simulink model "SI_Model_Manual"  (R2017b)
settings: Solver=VariableStepAuto  StartTime=0.0  StopTime=500  RelTol=1e-3
model workspace (MAT data in the model file):
  DOWN_TABLE = [0  5  20  35; 0  5  20  35; 0  5  25  40; 0  5  30  50; 0  30  50  80; 0  30  50  80]
  DOWN_TH_BP = [0; 0.05; 0.4; 0.5; 0.9; 1]
  TWAIT = 2
  UP_TABLE = [10  30  50  1000000; 10  30  50  1000000; 15  30  50  1000000; 23  41  60  1000000; 40  70  100  1000000; 40  70  100  1000000]
  UP_TH_BP = [0; 0.25; 0.35; 0.5; 0.9; 1]
  Var1 = 0
  clutchRise = 0.1
  eff_tor_rad = 0.4
  engagement_area = 0.0025
  fric_coeff = 0.5
  gear1 = 3.07
  gear2 = 1.913
  gear3 = 1.258
  gear4 = 0.943
  gear5 = 0.763
  gearx = 4.529
  num_fric_surf = 6
  p0 = 2000000
  peak_normal = 0.55
  pressThresh = 0.05
  v0 = 0
  velTol = 0.001
values from neighbouring files (symbols this model uses):
  HEV_Param =     [DataWorkSpace.mat]
libraries: sdl_lib x17, nesl_utility x15, fl_lib x13, drivecyclelib x1, simulink x1
settings Model: PauseTimes=60  Creator=Charlie  LastModifiedBy=Charlie
settings SolverCC: ZeroCrossAlgorithm=Adaptive  AlgebraicLoopSolver=LineSearch
settings SimscapeCC: SimscapeLogType=all  SimscapeLogSimulationStatistics=on  SimscapeLogOpenViewer=on

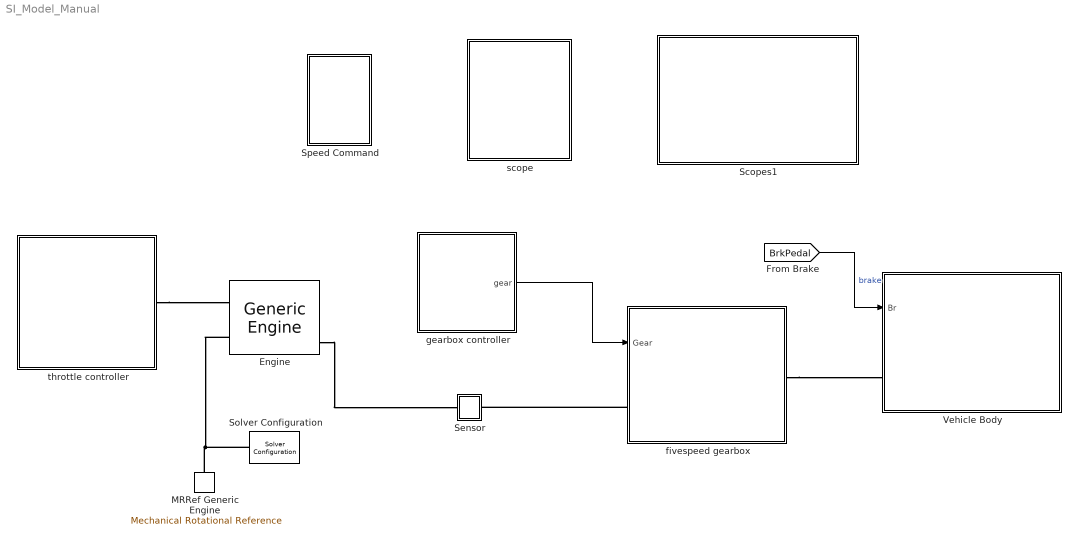
== system SI_Model_Manual ==
  Engine : sdl_lib/Engines/Generic Engine  model_parameterization=1  engine_type=1  P_max=52 kW  w_P_max=6000 rpm  w_max=7000 rpm  w_min=500 rpm  w_tab=[ 500 1000 2e+3 3e+3 4e+3 5e+3 6e+3 7e+3 ] rpm  trq_tab=[ 40 41 42 46 49 42 41 40 ] N*m  pwr_tab=[ 2e+4 4e+4 7.8e+4 1.2e+5 1.45e+5 1.48e+5 1.25e+5 6e+4 ] W  interp_method=1  model_inertia=1  inertia=HEV_Param.ICE.Shaft_Inertia kg*m^2  initial_velocity=800 rpm  model_time_constant=1  time_constant=0.01 s  T0=0  w_thr=100 rpm  idle_speed=1  idle_speed_reference=800 rpm  tau_controller=0.01 s  idle_w_thr=1 rpm  redline=0  redline_speed=7000 rpm  tau_redline=1 s  redline_w_thr=1 rpm  fc_model=1  fc_per_rev=6.2 mg/rev  displaced_volume=400 cm^3  rev_per_cycle=2  fc_w_tab=[ 1000 2e+3 3e+3 4e+3 5e+3 6e+3 ] rpm  fc_trq_tab=[ 0 80 160 200 240 320 360 400 ] N*m  fc_tab=[ 0.5 0.9 1.4 1.6 1.9 2.7 3.4 4.4; 1 1.7 2.7 3.1 3.6 5 6 7.4; 1.4 2.7 4 4.8 5.6 7.5 8.5 10.5; 2 3.6 5.8 6.7 8 10.4 11.7 13.3; 2.5 4.8 7.9 9.4 10.8 14 16.2 18.6; 3.1 6 10.3 11.9 13.8 18.4 22 26.5 ] g/s  bmep_tab=[ 0 250 500 625 750 1000 1.15e+3 1.25e+3 ] kPa  bsfc_tab=[ 410 380 300 280 270 290 320 380; 410 370 290 270 260 270 285 320; 415 380 290 275 265 270 270 300; 420 390 310 290 285 280 280 285; 430 410 340 320 310 300 310 320; 450 430 370 340 330 330 350 380 ] g/hr/kW  fc_interp_method=1
      settings: SourceProductName=Simscape Driveline  SourceProductBaseCode=LD
  MRRef Generic Engine : fl_lib/Mechanical/Rotational Elements/Mechanical Rotational Reference
  Scopes1 : Subsystem  mask(Data Acquisition){}
      mask Display: image('D:\Matlab\Powertrain\Plot\Fuel_Tank.jpg');
  Sensor : Subsystem
      mask Display: disp('S');
  Solver Configuration : nesl_utility/Solver Configuration  PhysicalDomain=network_engine_domain  SubClassName=solver  LeftPortType=input  RightPortType=generic  Accelerate=off  Tones=[]  Harmonics=[]  SimulateNoise=off  Profile=off  UseLocalSampling=off  EnableSwitchedLinearOptims=on  FrequencyDomain=off  UseCCode=off  RelTol=0.001  AbsTol=1e-06  MinStep=1e-09  ToWorkspace=off  RevertToSquareIcSolve=off  NumHomotopyIterations=100  PhasorMode=off  PhasorModeNumHarmonics=1  DoDC=off  ResidualTolerance=1e-9  UseLocalSolver=off  LocalSolverChoice=NE_BACKWARD_EULER_ADVANCER  LocalSolverSampleTime=.01  DoFixedCost=off  MaxNonlinIter=3  MaxModeIter=2  LinearAlgebra=Sparse  DelaysMemoryBudget=1024  AutomaticFiltering=on  FilteringTimeConstant=0.001
  Speed Command : Subsystem
  Vehicle Body : Subsystem  Tag=PublishSubsystem
      mask Display: image('D:\Matlab\Powertrain\Plot\smart_fortw.jpg');
  fivespeed gearbox : Subsystem  Tag=PublishSubsystem
      mask Display: image(imread('sdl_transmission_5spd_schematic.jpg'),'center');
  gearbox controller : Subsystem
  scope : Subsystem
  throttle controller : Subsystem
      mask Display: image('D:\Matlab\Powertrain\Plot\throttle.JPG');
  wires:
  [BrkPedal] -> Vehicle Body/1(Br)  "brake"
  gearbox controller/1(gear) -> fivespeed gearbox/1(Gear)
  connections:
  MRRef Generic Engine/LConn1 -- Engine/LConn2 -- Solver Configuration/RConn1
  fivespeed gearbox/LConn1 -- Sensor/RConn1
  fivespeed gearbox/RConn1 -- Vehicle Body/LConn1
  Engine/RConn3 -- Sensor/LConn1
  throttle controller/RConn1 -- Engine/LConn1

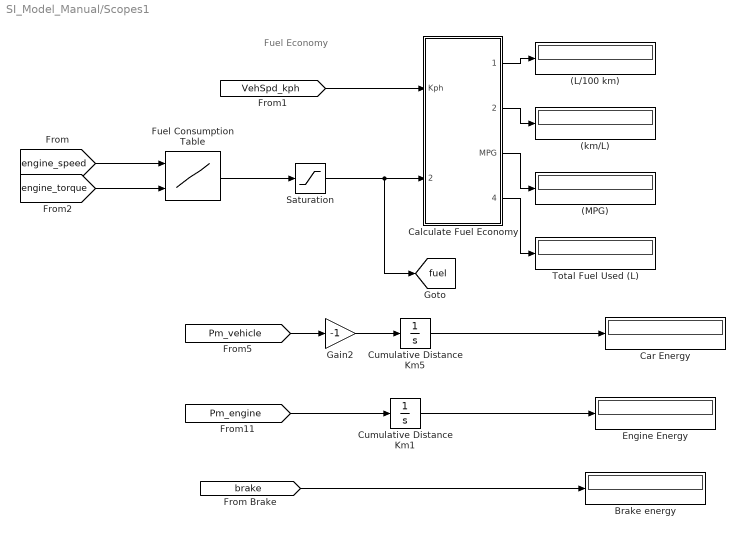
== system SI_Model_Manual/Scopes1 ==
  note: Fuel Economy
  (L/100 km) : Display
      settings: Decimation=decimation
  (MPG) : Display
      settings: Decimation=decimation
  (km/L) : Display
      settings: Decimation=decimation
  Brake energy : Display
      settings: Decimation=decimation
  Calculate Fuel Economy : Subsystem
  Car Energy : Display
      settings: Decimation=decimation
  Cumulative Distance Km1 : Integrator  InitialCondition=eps
  Cumulative Distance Km5 : Integrator  InitialCondition=eps
  Engine Energy : Display
      settings: Decimation=decimation
  Fuel Consumption Table : Lookup2D  RowIndex=HEV_Param.ICE.FC.Speed_Vector  ColumnIndex=HEV_Param.ICE.FC.Torque_Vector  Table=HEV_Param.ICE.FC.Consumption_Table
  Gain2 : Gain  Gain=-1
  Saturation : Saturate  UpperLimit=inf  LowerLimit=0
  Total Fuel Used (L) : Display
      settings: Decimation=decimation
  tag scope: fuel=global
  wires:
  Calculate Fuel Economy/1(Liter/100Km) -> (L/100 km)/1
  Calculate Fuel Economy/3(MPG) -> (MPG)/1
  [VehSpd_kph] -> Calculate Fuel Economy/1(Kph)
  Calculate Fuel Economy/4(Fuel Used (L)) -> Total Fuel Used (L)/1
  Calculate Fuel Economy/2(Km/Liter) -> (km/L)/1
  Fuel Consumption Table/1 -> Saturation/1
  [engine_speed] -> Fuel Consumption Table/1
  [engine_torque] -> Fuel Consumption Table/2
  Gain2/1 -> Cumulative Distance Km5/1
  Cumulative Distance Km5/1 -> Car Energy/1
  [Pm_vehicle] -> Gain2/1
  [Pm_engine] -> Cumulative Distance Km1/1
  Cumulative Distance Km1/1 -> Engine Energy/1
  [brake] -> Brake energy/1
  Saturation/1 -> [fuel], Calculate Fuel Economy/2(Fuel Flow g/s)

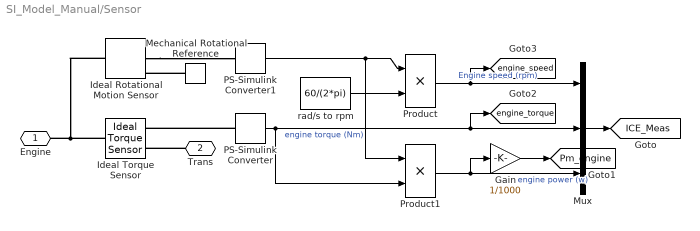
== system SI_Model_Manual/Sensor ==
  Gain : Gain  Gain=1/1000
  Ideal Rotational Motion Sensor : fl_lib/Mechanical/Mechanical Sensors/Ideal Rotational Motion Sensor  offset=0 rad
  Ideal Torque Sensor : fl_lib/Mechanical/Mechanical Sensors/Ideal Torque Sensor
  Mechanical Rotational Reference : fl_lib/Mechanical/Rotational Elements/Mechanical Rotational Reference
  Mux : Mux  Inputs=3
  PS-Simulink Converter : nesl_utility/PS-Simulink Converter  PhysicalDomain=network_engine_domain  SubClassName=ps_output  LeftPortType=input  RightPortType=output  PseudoPeriodic=off  Frequencies=[]  Unit=N*m  AffineConversion=off
  PS-Simulink Converter1 : nesl_utility/PS-Simulink Converter  PhysicalDomain=network_engine_domain  SubClassName=ps_output  LeftPortType=input  RightPortType=output  PseudoPeriodic=off  Frequencies=[]  Unit=rad/s  AffineConversion=off
  Product : Product  RndMeth=Zero
  Product1 : Product  RndMeth=Zero
  rad/s to rpm : Constant  Value=60/(2*pi)
  Engine : PMIOPort  Port=1  Side=Left
  Trans : PMIOPort  Port=2  Side=Right
  tag scope: ICE_Meas=global, Pm_engine=global, engine_speed=global, engine_torque=global
  wires:
  PS-Simulink Converter/1 -> Product1/2, Mux/2, [engine_torque]  "engine torque (Nm)"
  Product1/1 -> Gain/1, Mux/3  "engine power (w)"
  Product/1 -> Mux/1, [engine_speed]  "Engine speed (rpm)"
  PS-Simulink Converter1/1 -> Product/1, Product1/1
  rad/s to rpm/1 -> Product/2
  Mux/1 -> [ICE_Meas]
  Gain/1 -> [Pm_engine]
  connections:
  Ideal Torque Sensor/LConn1 -- Engine/RConn1 -- Ideal Rotational Motion Sensor/LConn1
  Trans/RConn1 -- Ideal Torque Sensor/RConn1
  PS-Simulink Converter/LConn1 -- Ideal Torque Sensor/RConn2
  Ideal Rotational Motion Sensor/RConn2 -- PS-Simulink Converter1/LConn1
  Mechanical Rotational Reference/LConn1 -- Ideal Rotational Motion Sensor/RConn1

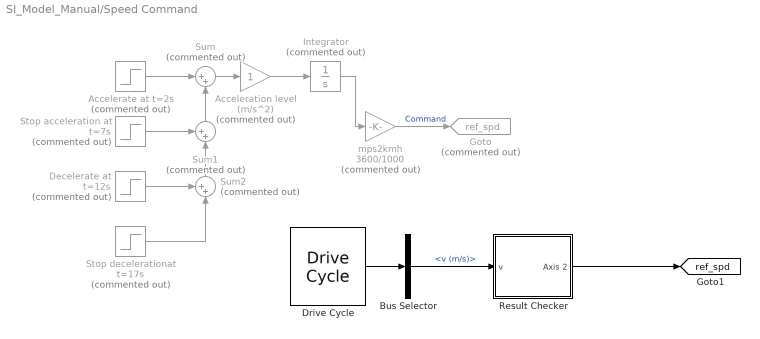
== system SI_Model_Manual/Speed Command ==
  Accelerate at t=2s : Step  Commented=on  Time=2  SampleTime=0
  Acceleration level (m/s^2) : Gain  Commented=on
  Bus Selector : BusSelector  OutputSignals=v (m/s)
  Decelerate at t=12s : Step  Commented=on  Time=12  After=-1  SampleTime=0
  Drive Cycle : drivecyclelib/Drive Cycle  CycleName=ECE R15  CycleRepeatsForever=off
      settings: SourceProductName=Drive Cycles Blockset
  Goto : Goto  Commented=on  GotoTag=ref_spd  TagVisibility=global
  Integrator : Integrator  Commented=on  InitialCondition=v0
  Result Checker : Subsystem
  Stop acceleration at t=7s : Step  Commented=on  Time=7  After=-1  SampleTime=0
  Stop decelerationat t=17s : Step  Commented=on  Time=17  SampleTime=0
  Sum : Sum  Commented=on  Inputs=|++
  Sum1 : Sum  Commented=on  Inputs=++|
  Sum2 : Sum  Commented=on  Inputs=++|
  mps2kmh : Gain  Commented=on  Gain=3600/1000
  tag scope: ref_spd=global
  wires:
  mps2kmh/1 -> Goto/1  "Command"
  Stop decelerationat t=17s/1 -> Sum2/2
  Decelerate at t=12s/1 -> Sum2/1
  Acceleration level (m/s^2)/1 -> Integrator/1
  Sum2/1 -> Sum1/2
  Sum1/1 -> Sum/2
  Stop acceleration at t=7s/1 -> Sum1/1
  Integrator/1 -> mps2kmh/1
  Sum/1 -> Acceleration level (m/s^2)/1
  Accelerate at t=2s/1 -> Sum/1
  Drive Cycle/1 -> Bus Selector/1
  Bus Selector/1 -> Result Checker/1(v)  "<v (m/s)>"
  Result Checker/1(Axis 2) -> [ref_spd]

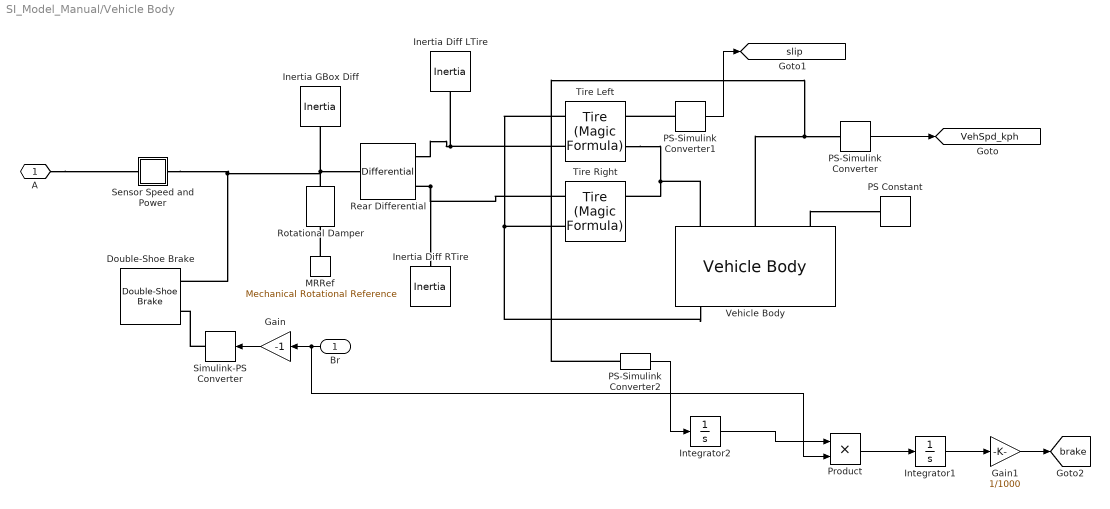
== system SI_Model_Manual/Vehicle Body ==
  Br : Inport
  Double-Shoe Brake : sdl_lib/Brakes & Detents/Rotational/Double-Shoe Brake  r_drum=200 mm  r_act=100 mm  r_pin=125 mm  theta_pin=15 deg  theta_0=5 deg  theta_shoe=120 deg  mu_visc=.01 N*m/(rad/s)  mu=0.38  w_thr=0.01 rad/s  temperature_TLU=[280, 300, 320] K  mu_TLU=[.1, .05, .03]  thermal_mass=50 kJ/K  temperature_specify=off  temperature_priority=High  temperature=300 K  temperature_nominal_specify=off  temperature_nominal_unit=K  temperature_nominal_value=1
      settings: SourceProductName=Simscape Driveline  SourceProductBaseCode=LD
  Gain : Gain  Gain=-1
  Gain1 : Gain  Gain=1/1000
  Inertia Diff LTire : fl_lib/Mechanical/Rotational Elements/Inertia  inertia=HEV_Param.Vehicle.Wheel_Inertia*2 kg*m^2  w_specify=on  w_priority=High  w=v0/HEV_Param.Vehicle.Tire_Radius rad/s  w_nominal_specify=off  w_nominal_unit=rad/s  w_nominal_value=1  t_specify=off  t_priority=High  t=0 N*m  t_nominal_specify=off  t_nominal_unit=N*m  t_nominal_value=1
  Inertia Diff RTire : fl_lib/Mechanical/Rotational Elements/Inertia  inertia=HEV_Param.Vehicle.Wheel_Inertia*2 kg*m^2  w_specify=on  w_priority=High  w=v0/HEV_Param.Vehicle.Tire_Radius rad/s  w_nominal_specify=off  w_nominal_unit=rad/s  w_nominal_value=1  t_specify=off  t_priority=High  t=0 N*m  t_nominal_specify=off  t_nominal_unit=N*m  t_nominal_value=1
  Inertia GBox Diff : fl_lib/Mechanical/Rotational Elements/Inertia  inertia=HEV_Param.Vehicle.Trans.Inertia kg*m^2  w_specify=on  w_priority=High  w=v0/HEV_Param.Vehicle.Tire_Radius rad/s  w_nominal_specify=off  w_nominal_unit=rad/s  w_nominal_value=1  t_specify=off  t_priority=High  t=0 N*m  t_nominal_specify=off  t_nominal_unit=N*m  t_nominal_value=1
  Integrator1 : Integrator
  Integrator2 : Integrator
  MRRef : fl_lib/Mechanical/Rotational Elements/Mechanical Rotational Reference
  PS Constant : fl_lib/Physical Signals/Sources/PS Constant  constant=5
  PS-Simulink Converter : nesl_utility/PS-Simulink Converter  PhysicalDomain=network_engine_domain  SubClassName=ps_output  LeftPortType=input  RightPortType=output  PseudoPeriodic=off  Frequencies=[]  Unit=km/hr  AffineConversion=off
  PS-Simulink Converter1 : nesl_utility/PS-Simulink Converter  PhysicalDomain=network_engine_domain  SubClassName=ps_output  LeftPortType=input  RightPortType=output  PseudoPeriodic=off  Frequencies=[]  Unit=km/hr  AffineConversion=off
  PS-Simulink Converter2 : nesl_utility/PS-Simulink Converter  PhysicalDomain=network_engine_domain  SubClassName=ps_output  LeftPortType=input  RightPortType=output  PseudoPeriodic=off  Frequencies=[]  Unit=m/s  AffineConversion=off
  Product : Product
  Rear Differential : sdl_lib/Gears/Differential  driveshaft_location=2  cd_ratio=1  friction_model=1  efficiency=[ 0.85 0.92 ]  mu_visc=[ 0 0 ] N*m/(rad/s)  pwr_thr=[ 0.001 0.001 ] W  carrier_inertia=0 kg*m^2  planet_inertia=0 kg*m^2  temperature_TLU=[ 280 300 320 ] K  efficiency_ss_TLU=[ 0.95 0.9 0.85 ]  efficiency_cd_TLU=[ 0.95 0.9 0.85 ]  thermal_mass=50 J/K  T_init=300 K
      settings: SourceProductName=Simscape Driveline  SourceProductBaseCode=LD
  Rotational Damper : fl_lib/Mechanical/Rotational Elements/Rotational Damper  D=HEV_Param.Vehicle.Trans.Friction N*m/(rad/s)  w_specify=on  w_priority=High  w=v0/HEV_Param.Vehicle.Tire_Radius rad/s  w_nominal_specify=off  w_nominal_unit=rad/s  w_nominal_value=1  t_specify=off  t_priority=High  t=0 N*m  t_nominal_specify=off  t_nominal_unit=N*m  t_nominal_value=1
  Sensor Speed and Power : Subsystem
      mask Display: disp('S')
  Simulink-PS Converter : nesl_utility/Simulink-PS Converter  PhysicalDomain=network_engine_domain  SubClassName=ps_input  LeftPortType=input  RightPortType=output  PseudoPeriodic=off  Frequencies=[]  NoiseDistribution=none  NoiseParameters=[]  Unit=1  AffineConversion=off  FilteringAndDerivatives=zero  SimscapeFilterOrder=1  InputFilterTimeConstant=0.001  UdotUserProvided=1
  Tire Left : sdl_lib/Tires & Vehicles/Tire (Magic Formula)  parameterization=1  F_z1=HEV_Param.Vehicle.Tire.Rated_Vertical_Load N  F_x1=HEV_Param.Vehicle.Tire.Rated_Peak_Long_Force N  kappa1=HEV_Param.Vehicle.Tire.Slip_At_Peak_Force  B_m=10  C_m=1.9  D_m=1  E_m=0.97  fz0=4e+3 N  p_Cx=1.685  p_Dx=[ 1.21 -0.037 ]  p_Ex=[ 0.344 0.095 -0.02 0 ]  p_Kx=[ 21.51 -0.163 0.245 ]  p_Hx=[ -0.002 0.002 ]  p_Vx=[ 0 0 ]  v_tr_thr=0.1 m/s  r_e=HEV_Param.Vehicle.Tire_Radius m  model_compliance=0  stiffness=1e+6 N/m  damping=1000 N/(m/s)  model_inertia=1  inertia=1e-2 kg*m^2  initial_velocity=v0/HEV_Param.Vehicle.Tire_Radius rad/s  model_resistance=0  resistance_model=1  coeff=0.015  p_tire=2.5e+5 Pa  alpha=-0.003  beta=0.97  coeff_a=0.008399999999999999  coeff_b=6.2e-4 s/m  coeff_c=1.6e-4 s^2/m^2  v_thr=0.001 m/s
      settings: SourceProductName=Simscape Driveline
  Tire Right : sdl_lib/Tires & Vehicles/Tire (Magic Formula)  parameterization=1  F_z1=HEV_Param.Vehicle.Tire.Rated_Vertical_Load N  F_x1=HEV_Param.Vehicle.Tire.Rated_Peak_Long_Force N  kappa1=HEV_Param.Vehicle.Tire.Slip_At_Peak_Force  B_m=10  C_m=1.9  D_m=1  E_m=0.97  fz0=4e+3 N  p_Cx=1.685  p_Dx=[ 1.21 -0.037 ]  p_Ex=[ 0.344 0.095 -0.02 0 ]  p_Kx=[ 21.51 -0.163 0.245 ]  p_Hx=[ -0.002 0.002 ]  p_Vx=[ 0 0 ]  v_tr_thr=0.1 m/s  r_e=HEV_Param.Vehicle.Tire_Radius m  model_compliance=0  stiffness=1e+6 N/m  damping=1000 N/(m/s)  model_inertia=1  inertia=1e-2 kg*m^2  initial_velocity=v0/HEV_Param.Vehicle.Tire_Radius rad/s  model_resistance=0  resistance_model=1  coeff=0.015  p_tire=2.5e+5 Pa  alpha=-0.003  beta=0.97  coeff_a=0.008399999999999999  coeff_b=6.2e-4 s/m  coeff_c=1.6e-4 s^2/m^2  v_thr=0.001 m/s
      settings: SourceProductName=Simscape Driveline
  Vehicle Body : sdl_lib/Tires & Vehicles/Vehicle Body  mass=HEV_Param.Vehicle.Mass kg  n_w=2  x_f=HEV_Param.Vehicle.Distance_CG_FrontAxle m  x_r=HEV_Param.Vehicle.Distance_CG_RearAxle m  y_c=HEV_Param.Vehicle.Distance_CG_Ground m  area=HEV_Param.Vehicle.Frontal_Area m^2  Cd=HEV_Param.Vehicle.Aero_Drag_Coeff  g=9.81 m/s^2  rho=1.18 kg/m^3  v_specify=on  v_priority=High  v=v0 m/s  v_nominal_specify=off  v_nominal_unit=m/s  v_nominal_value=1
      settings: SourceProductName=Simscape Driveline
  A : PMIOPort  Port=1  Side=Left
  tag scope: VehSpd_kph=global, brake=global, slip=global
  wires:
  PS-Simulink Converter/1 -> [VehSpd_kph]
  Gain/1 -> Simulink-PS Converter/1
  PS-Simulink Converter1/1 -> [slip]
  Integrator2/1 -> Product/1
  Gain1/1 -> [brake]
  Integrator1/1 -> Gain1/1
  PS-Simulink Converter2/1 -> Integrator2/1
  Br/1 -> Product/2, Gain/1
  Product/1 -> Integrator1/1
  connections:
  Tire Left/LConn1 -- Vehicle Body/RConn1 -- Tire Right/LConn1
  A/RConn1 -- Sensor Speed and Power/LConn1
  Tire Left/RConn2 -- Vehicle Body/LConn1 -- Tire Right/RConn2
  Vehicle Body/LConn2 -- PS-Simulink Converter2/LConn1 -- PS-Simulink Converter/LConn1
  Simulink-PS Converter/RConn1 -- Double-Shoe Brake/LConn1
  Vehicle Body/LConn3 -- PS Constant/RConn1
  Rear Differential/RConn1 -- Tire Right/LConn2 -- Inertia Diff RTire/LConn1
  Rear Differential/RConn2 -- Tire Left/LConn2 -- Inertia Diff LTire/LConn1
  MRRef/LConn1 -- Rotational Damper/RConn1
  PS-Simulink Converter1/LConn1 -- Tire Left/RConn1
  Sensor Speed and Power/RConn1 -- Rotational Damper/LConn1 -- Rear Differential/LConn1 -- Inertia GBox Diff/LConn1 -- Double-Shoe Brake/LConn2

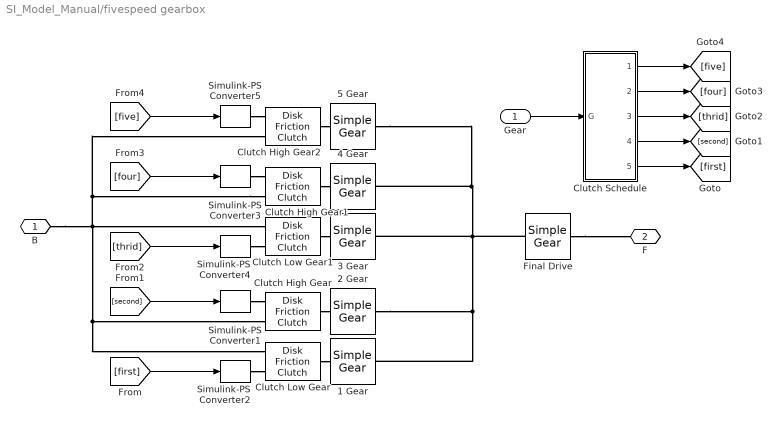
== system SI_Model_Manual/fivespeed gearbox ==
  Gear : Inport
  1 Gear : sdl_lib/Gears/Simple Gear  ratio=3.07  rotation_direction=2  friction_model=1  T_noload=0.1 N*m  T_nom=5 N*m  efficiency_nom=0.8  efficiency=0.98  mu_visc=[0 0] N*m/(rad/s)  w_thr=0.01 rad/s  pwr_thr=0.001 W  temperature_TLU=[ 280 300 320 ] K  load_TLU=[ 1 5 10 ] N*m  efficiency_TLU=[ 0.95 0.9 0.85 ]  efficiency_TLU2=[ 0.85 0.8 0.75; 0.95 0.9 0.85; 0.85 0.8 0.7 ]  thermal_mass=50 J/K  T_init=300 K
      settings: SourceProductName=Simscape Driveline
  2 Gear : sdl_lib/Gears/Simple Gear  ratio=1.913  rotation_direction=2  friction_model=1  T_noload=0.1 N*m  T_nom=5 N*m  efficiency_nom=0.8  efficiency=0.98  mu_visc=[ 0 0 ] N*m/(rad/s)  w_thr=0.01 rad/s  pwr_thr=0.001 W  temperature_TLU=[ 280 300 320 ] K  load_TLU=[ 1 5 10 ] N*m  efficiency_TLU=[ 0.95 0.9 0.85 ]  efficiency_TLU2=[ 0.85 0.8 0.75; 0.95 0.9 0.85; 0.85 0.8 0.7 ]  thermal_mass=50 J/K  T_init=300 K
      settings: SourceProductName=Simscape Driveline
  3 Gear : sdl_lib/Gears/Simple Gear  ratio=1.258  rotation_direction=2  friction_model=1  T_noload=0.1 N*m  T_nom=5 N*m  efficiency_nom=0.8  efficiency=0.98  mu_visc=[ 0 0 ] N*m/(rad/s)  w_thr=0.01 rad/s  pwr_thr=0.001 W  temperature_TLU=[ 280 300 320 ] K  load_TLU=[ 1 5 10 ] N*m  efficiency_TLU=[ 0.95 0.9 0.85 ]  efficiency_TLU2=[ 0.85 0.8 0.75; 0.95 0.9 0.85; 0.85 0.8 0.7 ]  thermal_mass=50 J/K  T_init=300 K
      settings: SourceProductName=Simscape Driveline
  4 Gear : sdl_lib/Gears/Simple Gear  ratio=0.943  rotation_direction=2  friction_model=2  T_noload=0.1 N*m  T_nom=5 N*m  efficiency_nom=0.8  efficiency=0.98  mu_visc=[ 0.02 0.02 ] N*m/(rad/s)  w_thr=0.01 rad/s  pwr_thr=0.001 W  temperature_TLU=[ 280 300 320 ] K  load_TLU=[ 1 5 10 ] N*m  efficiency_TLU=[ 0.95 0.9 0.85 ]  efficiency_TLU2=[ 0.85 0.8 0.75; 0.95 0.9 0.85; 0.85 0.8 0.7 ]  thermal_mass=50 J/K  T_init=300 K
      settings: SourceProductName=Simscape Driveline
  5 Gear : sdl_lib/Gears/Simple Gear  ratio=0.763  rotation_direction=2  friction_model=1  T_noload=0.1 N*m  T_nom=5 N*m  efficiency_nom=0.8  efficiency=0.8  mu_visc=[ 0 0 ] N*m/(rad/s)  w_thr=0.01 rad/s  pwr_thr=0.001 W  temperature_TLU=[ 280 300 320 ] K  load_TLU=[ 1 5 10 ] N*m  efficiency_TLU=[ 0.95 0.9 0.85 ]  efficiency_TLU2=[ 0.85 0.8 0.75; 0.95 0.9 0.85; 0.85 0.8 0.7 ]  thermal_mass=50 J/K  T_init=300 K
      settings: SourceProductName=Simscape Driveline
  Clutch High Gear : sdl_lib/Clutches/Disk Friction Clutch  geometry_model=1  r_eff=300 mm  d_o=150 mm  d_i=100 mm  nS=8  piston_area=0.001 m^2  unidirectional=0  friction_model=1  mu_coulomb=0.4  mu_w_vector=[ 0 0.1 0.2 0.3 0.4 0.5 1 2 5 10 100 1000 ] rad/s  mu_coulomb_vector=[ 0.29 0.28 0.26 0.22 0.21 0.2 0.2 0.19 0.19 0.19 0.19 0.19 ]  mu_interp_method=1  mu_extrap_method=1  mu_static=0.4  d_f=1  w_tol=0.001 rad/s  pressure_min=80 Pa  mu_visc=0 N*m/(rad/s)  initial_state_locked=0  temperature_TLU=[280.0, 300.0, 320.0] K  mu_coulomb_temp_vector=[0.3, 0.28, 0.25]  mu_coulomb_matrix=[0.34, 0.32, 0.3; 0.3, 0.28, 0.25; 0.25, 0.2, 0.15]  mu_static_vector=[0.4, 0.38, 0.36]  thermal_mass=25 kJ/K  T_init=300 K
      settings: SourceProductName=Simscape Driveline  SourceProductBaseCode=LD
  Clutch High Gear1 : sdl_lib/Clutches/Disk Friction Clutch  geometry_model=1  r_eff=300 mm  d_o=150 mm  d_i=100 mm  nS=4  piston_area=0.001 m^2  unidirectional=0  friction_model=1  mu_coulomb=0.4  mu_w_vector=[ 0 0.1 0.2 0.3 0.4 0.5 1 2 5 10 100 1000 ] rad/s  mu_coulomb_vector=[ 0.29 0.28 0.26 0.22 0.21 0.2 0.2 0.19 0.19 0.19 0.19 0.19 ]  mu_interp_method=1  mu_extrap_method=1  mu_static=0.4  d_f=1  w_tol=0.001 rad/s  pressure_min=80 Pa  mu_visc=0 N*m/(rad/s)  initial_state_locked=0  temperature_TLU=[280.0, 300.0, 320.0] K  mu_coulomb_temp_vector=[0.3, 0.28, 0.25]  mu_coulomb_matrix=[0.34, 0.32, 0.3; 0.3, 0.28, 0.25; 0.25, 0.2, 0.15]  mu_static_vector=[0.4, 0.38, 0.36]  thermal_mass=25 kJ/K  T_init=300 K
      settings: SourceProductName=Simscape Driveline  SourceProductBaseCode=LD
  Clutch High Gear2 : sdl_lib/Clutches/Disk Friction Clutch  geometry_model=1  r_eff=300 mm  d_o=150 mm  d_i=100 mm  nS=8  piston_area=0.001 m^2  unidirectional=0  friction_model=1  mu_coulomb=0.4  mu_w_vector=[ 0 0.1 0.2 0.3 0.4 0.5 1 2 5 10 100 1000 ] rad/s  mu_coulomb_vector=[ 0.29 0.28 0.26 0.22 0.21 0.2 0.2 0.19 0.19 0.19 0.19 0.19 ]  mu_interp_method=1  mu_extrap_method=1  mu_static=0.4  d_f=1  w_tol=0.001 rad/s  pressure_min=80 Pa  mu_visc=0 N*m/(rad/s)  initial_state_locked=0  temperature_TLU=[280.0, 300.0, 320.0] K  mu_coulomb_temp_vector=[0.3, 0.28, 0.25]  mu_coulomb_matrix=[0.34, 0.32, 0.3; 0.3, 0.28, 0.25; 0.25, 0.2, 0.15]  mu_static_vector=[0.4, 0.38, 0.36]  thermal_mass=25 kJ/K  T_init=300 K
      settings: SourceProductName=Simscape Driveline  SourceProductBaseCode=LD
  Clutch Low Gear : sdl_lib/Clutches/Disk Friction Clutch  geometry_model=1  r_eff=170 mm  d_o=150 mm  d_i=100 mm  nS=8  piston_area=0.001 m^2  unidirectional=0  friction_model=1  mu_coulomb=0.4  mu_w_vector=[ 0 0.1 0.2 0.3 0.4 0.5 1 2 5 10 100 1000 ] rad/s  mu_coulomb_vector=[ 0.29 0.28 0.26 0.22 0.21 0.2 0.2 0.19 0.19 0.19 0.19 0.19 ]  mu_interp_method=1  mu_extrap_method=1  mu_static=0.4  d_f=1  w_tol=0.001 rad/s  pressure_min=80 Pa  mu_visc=0 N*m/(rad/s)  initial_state_locked=0  temperature_TLU=[280.0, 300.0, 320.0] K  mu_coulomb_temp_vector=[0.3, 0.28, 0.25]  mu_coulomb_matrix=[0.34, 0.32, 0.3; 0.3, 0.28, 0.25; 0.25, 0.2, 0.15]  mu_static_vector=[0.4, 0.38, 0.36]  thermal_mass=25 kJ/K  T_init=300 K
      settings: SourceProductName=Simscape Driveline  SourceProductBaseCode=LD
  Clutch Low Gear1 : sdl_lib/Clutches/Disk Friction Clutch  geometry_model=1  r_eff=300 mm  d_o=150 mm  d_i=100 mm  nS=8  piston_area=0.001 m^2  unidirectional=0  friction_model=1  mu_coulomb=0.4  mu_w_vector=[ 0 0.1 0.2 0.3 0.4 0.5 1 2 5 10 100 1000 ] rad/s  mu_coulomb_vector=[ 0.29 0.28 0.26 0.22 0.21 0.2 0.2 0.19 0.19 0.19 0.19 0.19 ]  mu_interp_method=1  mu_extrap_method=1  mu_static=0.4  d_f=1  w_tol=0.001 rad/s  pressure_min=80 Pa  mu_visc=0 N*m/(rad/s)  initial_state_locked=0  temperature_TLU=[280.0, 300.0, 320.0] K  mu_coulomb_temp_vector=[0.3, 0.28, 0.25]  mu_coulomb_matrix=[0.34, 0.32, 0.3; 0.3, 0.28, 0.25; 0.25, 0.2, 0.15]  mu_static_vector=[0.4, 0.38, 0.36]  thermal_mass=25 kJ/K  T_init=300 K
      settings: SourceProductName=Simscape Driveline  SourceProductBaseCode=LD
  Clutch Schedule : Subsystem
  Final Drive : sdl_lib/Gears/Simple Gear  ratio=4.529  rotation_direction=2  friction_model=1  T_noload=0.1 N*m  T_nom=5 N*m  efficiency_nom=0.8  efficiency=0.98  mu_visc=[ 0 0] N*m/(rad/s)  w_thr=0.01 rad/s  pwr_thr=0.001 W  temperature_TLU=[ 280 300 320 ] K  load_TLU=[ 1 5 10 ] N*m  efficiency_TLU=[ 0.95 0.9 0.85 ]  efficiency_TLU2=[ 0.85 0.8 0.75; 0.95 0.9 0.85; 0.85 0.8 0.7 ]  thermal_mass=50 J/K  T_init=300 K
      settings: SourceProductName=Simscape Driveline
  Simulink-PS Converter{1..5} (5 alike) : nesl_utility/Simulink-PS Converter  PhysicalDomain=network_engine_domain  SubClassName=ps_input  LeftPortType=input  RightPortType=output  PseudoPeriodic=off  Frequencies=[]  NoiseDistribution=none  NoiseParameters=[]  Unit=Pa  AffineConversion=off  FilteringAndDerivatives=zero  SimscapeFilterOrder=1  InputFilterTimeConstant=.001  UdotUserProvided=0
  B : PMIOPort  Port=1  Side=Left
  F : PMIOPort  Port=2  Side=Right
  wires:
  Gear/1 -> Clutch Schedule/1(G)
  Clutch Schedule/5(1 Gear) -> [first]
  [first] -> Simulink-PS Converter2/1
  [second] -> Simulink-PS Converter1/1
  [thrid] -> Simulink-PS Converter4/1
  [four] -> Simulink-PS Converter3/1
  [five] -> Simulink-PS Converter5/1
  Clutch Schedule/1("5 Gear ") -> [five]
  Clutch Schedule/2(4 Gear) -> [four]
  Clutch Schedule/3(3 Gear) -> [thrid]
  Clutch Schedule/4("2 Gear ") -> [second]
  connections:
  Simulink-PS Converter1/RConn1 -- Clutch High Gear/LConn1
  Clutch Low Gear/RConn1 -- 1 Gear/LConn1
  Simulink-PS Converter2/RConn1 -- Clutch Low Gear/LConn1
  Clutch High Gear/RConn1 -- 2 Gear/LConn1
  Simulink-PS Converter4/RConn1 -- Clutch Low Gear1/LConn1
  Clutch High Gear1/RConn1 -- 4 Gear/LConn1
  Clutch Low Gear1/RConn1 -- 3 Gear/LConn1
  Simulink-PS Converter3/RConn1 -- Clutch High Gear1/LConn1
  2 Gear/RConn1 -- 5 Gear/RConn1 -- 4 Gear/RConn1 -- Final Drive/LConn1 -- 3 Gear/RConn1 -- 1 Gear/RConn1
  Clutch High Gear2/RConn1 -- 5 Gear/LConn1
  Simulink-PS Converter5/RConn1 -- Clutch High Gear2/LConn1
  Clutch High Gear1/LConn2 -- Clutch High Gear2/LConn2 -- Clutch Low Gear/LConn2 -- Clutch High Gear/LConn2 -- B/RConn1 -- Clutch Low Gear1/LConn2
  Final Drive/RConn1 -- F/RConn1

== system SI_Model_Manual/gearbox controller ==
  Chart : Stateflow chart  TreatAsAtomicUnit=on
  gear : Outport
  tag scope: gear=global
  wires:
  Chart/1(gear) -> gear/1, [gear]  "gear"
  [engine_speed] -> Chart/1(rpm)  "engine rpm"
  [ref_spd] -> Chart/3(RefSpeed)
  [VehSpd_kph] -> Chart/2(speed)

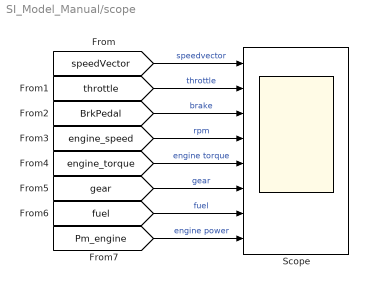
== system SI_Model_Manual/scope ==
  Scope : Scope  NumInputPorts=8
  wires:
  [speedVector] -> Scope/1  "speedvector"
  [throttle] -> Scope/2  "throttle"
  [BrkPedal] -> Scope/3  "brake"
  [engine_speed] -> Scope/4  "rpm"
  [engine_torque] -> Scope/5  "engine torque"
  [gear] -> Scope/6  "gear"
  [fuel] -> Scope/7  "fuel"
  [Pm_engine] -> Scope/8  "engine power"

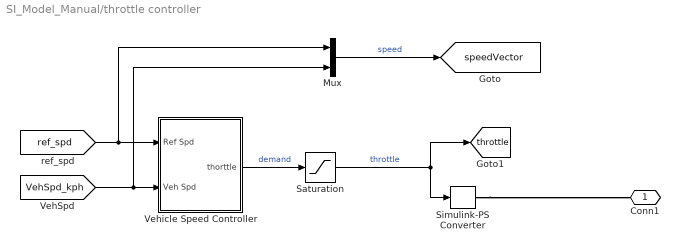
== system SI_Model_Manual/throttle controller ==
  Mux : Mux  Inputs=2
  Saturation : Saturate  UpperLimit=1  LowerLimit=0
  Simulink-PS Converter : nesl_utility/Simulink-PS Converter  PhysicalDomain=network_engine_domain  SubClassName=ps_input  LeftPortType=input  RightPortType=output  PseudoPeriodic=off  Frequencies=[]  NoiseDistribution=none  NoiseParameters=[]  Unit=1  AffineConversion=off  FilteringAndDerivatives=provide  SimscapeFilterOrder=1  InputFilterTimeConstant=0.001  UdotUserProvided=0
  Vehicle Speed Controller : Subsystem
  Conn1 : PMIOPort  Port=1  Side=Right
  tag scope: speedVector=global, throttle=global
  wires:
  Vehicle Speed Controller/1(thorttle) -> Saturation/1  "demand"
  [VehSpd_kph] -> Mux/2, Vehicle Speed Controller/2(Veh Spd)
  Saturation/1 -> Simulink-PS Converter/1, [throttle]  "throttle"
  [ref_spd] -> Mux/1, Vehicle Speed Controller/1(Ref Spd)
  Mux/1 -> [speedVector]  "speed"
  connections:
  Simulink-PS Converter/RConn1 -- Conn1/RConn1

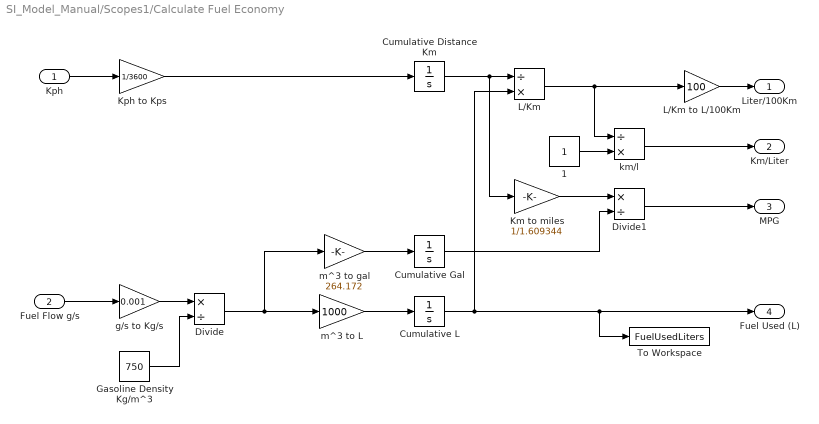
== system SI_Model_Manual/Scopes1/Calculate Fuel Economy ==
  Kph : Inport
  Fuel Flow g/s : Inport  Port=2
  1 : Constant
  Cumulative Distance Km : Integrator  InitialCondition=eps
  Cumulative Gal : Integrator  InitialCondition=eps
  Cumulative L : Integrator  InitialCondition=eps
  Divide : Product  Inputs=*/
  Divide1 : Product  Inputs=*/
  Gasoline Density Kg/m^3 : Constant  Value=750
  Km to miles : Gain  Gain=1/1.609344
  Kph to Kps : Gain  Gain=1/3600
  L/Km : Product  Inputs=/*
  L/Km to L/100Km : Gain  Gain=100
  To Workspace : ToWorkspace  VariableName=FuelUsedLiters  SampleTime=-1
      settings: MaxDataPoints=1
  g/s to Kg/s : Gain  Gain=0.001
  km/l : Product  Inputs=/*
  m^3 to L : Gain  Gain=1000
  m^3 to gal : Gain  Gain=264.172
  Liter/100Km : Outport
  Km/Liter : Outport  Port=2
  MPG : Outport  Port=3
  Fuel Used (L) : Outport  Port=4
  wires:
  km/l/1 -> Km/Liter/1
  1/1 -> km/l/2
  Divide1/1 -> MPG/1
  L/Km to L/100Km/1 -> Liter/100Km/1
  Fuel Flow g/s/1 -> g/s to Kg/s/1
  Kph/1 -> Kph to Kps/1
  Cumulative Gal/1 -> Divide1/2
  Km to miles/1 -> Divide1/1
  L/Km/1 -> km/l/1, L/Km to L/100Km/1
  Cumulative Distance Km/1 -> Km to miles/1, L/Km/1
  Cumulative L/1 -> L/Km/2, Fuel Used (L)/1, To Workspace/1
  Kph to Kps/1 -> Cumulative Distance Km/1
  m^3 to gal/1 -> Cumulative Gal/1
  m^3 to L/1 -> Cumulative L/1
  Divide/1 -> m^3 to gal/1, m^3 to L/1
  Gasoline Density Kg/m^3/1 -> Divide/2
  g/s to Kg/s/1 -> Divide/1

== system SI_Model_Manual/Speed Command/Result Checker ==
  v : Inport
  m/s to km/h : Gain  Gain=3.6
  Axis 2 : Outport
  wires:
  v/1 -> m/s to km/h/1
  m/s to km/h/1 -> Axis 2/1  "v, integral of a (km/h)"

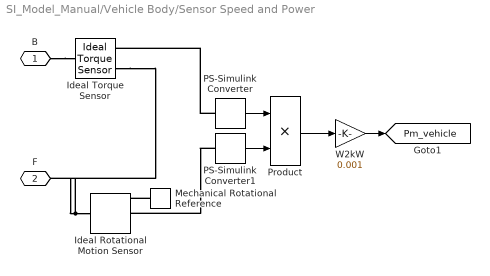
== system SI_Model_Manual/Vehicle Body/Sensor Speed and Power ==
  Ideal Rotational Motion Sensor : fl_lib/Mechanical/Mechanical Sensors/Ideal Rotational Motion Sensor  offset=0 rad
  Ideal Torque Sensor : fl_lib/Mechanical/Mechanical Sensors/Ideal Torque Sensor
  Mechanical Rotational Reference : fl_lib/Mechanical/Rotational Elements/Mechanical Rotational Reference
  PS-Simulink Converter : nesl_utility/PS-Simulink Converter  PhysicalDomain=network_engine_domain  SubClassName=ps_output  LeftPortType=input  RightPortType=output  PseudoPeriodic=off  Frequencies=[]  Unit=N*m  AffineConversion=off
  PS-Simulink Converter1 : nesl_utility/PS-Simulink Converter  PhysicalDomain=network_engine_domain  SubClassName=ps_output  LeftPortType=input  RightPortType=output  PseudoPeriodic=off  Frequencies=[]  Unit=rad/s  AffineConversion=off
  Product : Product  RndMeth=Zero
  W2kW : Gain  Gain=0.001
  B : PMIOPort  Port=1  Side=Left
  F : PMIOPort  Port=2  Side=Right
  tag scope: Pm_vehicle=global
  wires:
  W2kW/1 -> [Pm_vehicle]
  Product/1 -> W2kW/1
  PS-Simulink Converter/1 -> Product/1
  PS-Simulink Converter1/1 -> Product/2
  connections:
  Mechanical Rotational Reference/LConn1 -- Ideal Rotational Motion Sensor/RConn1
  Ideal Rotational Motion Sensor/LConn1 -- F/RConn1 -- Ideal Torque Sensor/RConn1
  B/RConn1 -- Ideal Torque Sensor/LConn1
  PS-Simulink Converter/LConn1 -- Ideal Torque Sensor/RConn2
  PS-Simulink Converter1/LConn1 -- Ideal Rotational Motion Sensor/RConn2

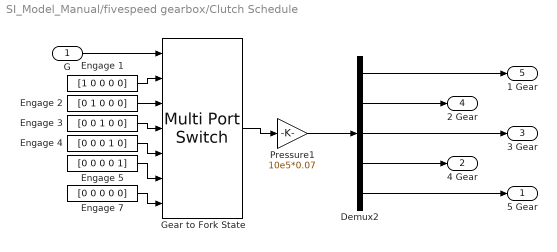
== system SI_Model_Manual/fivespeed gearbox/Clutch Schedule ==
  G : Inport
  Demux2 : Demux  Outputs=5
  Engage 1 : Constant  Value=[1 0 0 0 0]
  Engage 2 : Constant  Value=[0 1 0 0 0]
  Engage 3 : Constant  Value=[0 0 1 0 0]
  Engage 4 : Constant  Value=[0 0 0 1 0]
  Engage 5 : Constant  Value=[0 0 0 0 1]
  Engage 7 : Constant  Value=[0 0 0 0 0]
  Gear to Fork State : MultiPortSwitch  DataPortOrder=Specify indices  DataPortIndices={1,2,3,4,5,0}  DiagnosticForDefault=None
  Pressure1 : Gain  Gain=10e5*0.07  SaturateOnIntegerOverflow=on  OutDataTypeStr=Inherit: Same as input  ParamDataTypeStr=Inherit: Same as input
  "5 Gear " : Outport
  4 Gear : Outport  Port=2
  3 Gear : Outport  Port=3
  "2 Gear " : Outport  Port=4
  1 Gear : Outport  Port=5
  wires:
  G/1 -> Gear to Fork State/1
  Engage 4/1 -> Gear to Fork State/5
  Engage 1/1 -> Gear to Fork State/2
  Engage 2/1 -> Gear to Fork State/3
  Engage 7/1 -> Gear to Fork State/7
  Engage 5/1 -> Gear to Fork State/6
  Engage 3/1 -> Gear to Fork State/4
  Gear to Fork State/1 -> Pressure1/1
  Pressure1/1 -> Demux2/1
  Demux2/5 -> "5 Gear "/1
  Demux2/4 -> 4 Gear/1
  Demux2/3 -> 3 Gear/1
  Demux2/2 -> "2 Gear "/1
  Demux2/1 -> 1 Gear/1

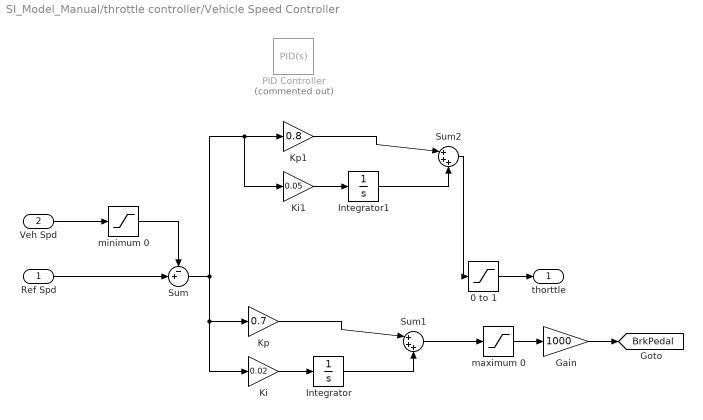
== system SI_Model_Manual/throttle controller/Vehicle Speed Controller ==
  Ref Spd : Inport
  Veh Spd : Inport  Port=2
  0 to 1 : Saturate  UpperLimit=0.6  LowerLimit=0
  Gain : Gain  Gain=1000
  Integrator : Integrator
  Integrator1 : Integrator
  Ki : Gain  Gain=0.02
  Ki1 : Gain  Gain=0.05
  Kp : Gain  Gain=0.7
  Kp1 : Gain  Gain=0.8
  PID Controller : simulink/Continuous/PID Controller  Commented=on  Controller=PID  TimeDomain=Continuous-time  SampleTime=-1  IntegratorMethod=Forward Euler  FilterMethod=Forward Euler  Form=Parallel  UseFilter=on  ControllerParametersSource=internal  P=0.4  I=0.11  D=0.1  N=100  InitialConditionSource=internal  InitialConditionForIntegrator=0  InitialConditionForFilter=0  ExternalReset=none  LimitOutput=off  UpperSaturationLimit=inf  LowerSaturationLimit=-inf  LinearizeAsGain=on  AntiWindupMode=none  Kb=1  TrackingMode=off  Kt=1  PParamMin=[]  PParamMax=[]  IParamMin=[]  IParamMax=[]  DParamMin=[]  DParamMax=[]  NParamMin=[]  NParamMax=[]  KbParamMin=[]  KbParamMax=[]  KtParamMin=[]  KtParamMax=[]  POutMin=[]  POutMax=[]  IOutMin=[]  IOutMax=[]  DOutMin=[]  DOutMax=[]  NOutMin=[]  NOutMax=[]  KbOutMin=[]  KbOutMax=[]  KtOutMin=[]  KtOutMax=[]  IntegratorOutMin=[]  IntegratorOutMax=[]  FilterOutMin=[]  FilterOutMax=[]  SumOutMin=[]  SumOutMax=[]  SumI1OutMin=[]  SumI1OutMax=[]  SumI2OutMin=[]  SumI2OutMax=[]  SumI3OutMin=[]  SumI3OutMax=[]  SumDOutMin=[]  SumDOutMax=[]  SaturationOutMin=[]  SaturationOutMax=[]  IntegratorContinuousStateAttributes=''  IntegratorStateMustResolveToSignalObject=off  IntegratorRTWStateStorageClass=Auto  FilterContinuousStateAttributes=''  FilterStateMustResolveToSignalObject=off  FilterRTWStateStorageClass=Auto  DifferentiatorICPrevScaledInput=0  DifferentiatorOutMin=[]  DifferentiatorOutMax=[]  InitialConditionSetting=State (most efficient)  FilterDiffOutCoefMin=[]  FilterDiffOutCoefMax=[]  SumDenOutMin=[]  SumDenOutMax=[]  SumNumOutMin=[]  SumNumOutMax=[]  ReciprocalOutMin=[]  ReciprocalOutMax=[]  DivideOutMin=[]  DivideOutMax=[]  TunerSelectOption=Transfer Function Based (PID Tuner App)
  Sum : Sum  Inputs=-+|
  Sum1 : Sum  Inputs=|+++
  Sum2 : Sum  Inputs=|+++
  maximum 0 : Saturate  UpperLimit=0  LowerLimit=-inf
  minimum 0 : Saturate  UpperLimit=inf  LowerLimit=0
  thorttle : Outport
  tag scope: BrkPedal=global
  wires:
  0 to 1/1 -> thorttle/1
  Ref Spd/1 -> Sum/2
  Veh Spd/1 -> minimum 0/1
  Sum2/1 -> 0 to 1/1
  Gain/1 -> [BrkPedal]
  maximum 0/1 -> Gain/1
  Sum1/1 -> maximum 0/1
  Integrator/1 -> Sum1/3
  Kp/1 -> Sum1/1
  Ki/1 -> Integrator/1
  minimum 0/1 -> Sum/1
  Integrator1/1 -> Sum2/3
  Ki1/1 -> Integrator1/1
  Kp1/1 -> Sum2/1
  Sum/1 -> Ki1/1, Kp1/1, Ki/1, Kp/1

== stateflow chart SI_Model_Manual/gearbox controller/Chart ==
  settings: stateMachineType=MOORE_MACHINE
  state first
    gear=1;
  state netural
    gear=0;
  state second
    gear=2;
  state fifth
    gear=5;
  state third
    gear=3;
  state fourth
    gear=4;
  first -> second [order 1] : [(RefSpeed>0)&&(speed>15)&&(rpm>2500)]
  netural -> first : [RefSpeed>0]
  second -> first [order 1] : [(RefSpeed<=0)||(speed<10)&&(rpm<1600)]
  first -> netural [order 2] : [[RefSpeed<=0] ]
  (default) -> netural
  second -> third [order 2] : [(RefSpeed>0)&&(speed>38)&&(rpm>2500)&&after(10,sec)]
  third -> second [order 1] : [(RefSpeed<=0)||(speed<22)||(rpm<2000)]
  fourth -> fifth [order 2] : [(RefSpeed>0)&&(speed>115)&&(rpm>5700) ]
  fifth -> fourth : [(RefSpeed<=0)||(speed<60)||(rpm<2000)]
  fourth -> third [order 1] : [(RefSpeed<=0)||(speed<40)||(rpm<2000)]
  third -> fourth [order 2] : [(RefSpeed>0)&&(speed>100)&&(rpm>5300)&&after(20,sec) ]
  data: rpm input; speed input; RefSpeed input; gear output
